simulink model "Ejercicio_2_DB"  (R2023a)
settings: Solver=VariableStepAuto  StartTime=0.0  StopTime=.5  RelTol=1e-6
values from neighbouring files (symbols this model uses):
  C3 = 10e-6    (= 1e-05)    [Ejercicio_2.m]
  C5 = C3    (= 1e-05)    [Ejercicio_2.m]
  G0 = 1/(C*inv(B*K-A)*B)    [Ejercicio_2.m]
  G1 = 1/R1    (= 0.001)    [Ejercicio_2.m]
  G2 = 1/R2    (= 0.001)    [Ejercicio_2.m]
  G4 = 1/R4    (= 0.0005)    [Ejercicio_2.m]
  G6a = 1/R6a    (= 0.001)    [Ejercicio_2.m]
  G6b = 1/R6b    (= 0.001)    [Ejercicio_2.m]
  K = acker(A,B,P_LC)    [Ejercicio_2.m]
settings Model: Creator=54115  LastModifiedBy=franc
settings SolverCC: AlgebraicLoopSolver=TrustRegion
settings DebuggingCC: UnconnectedInputMsg=warning  UnconnectedOutputMsg=warning  UnconnectedLineMsg=warning
settings ModelReferenceCC: EnableRefExpFcnMdlSchedulingChecks=on

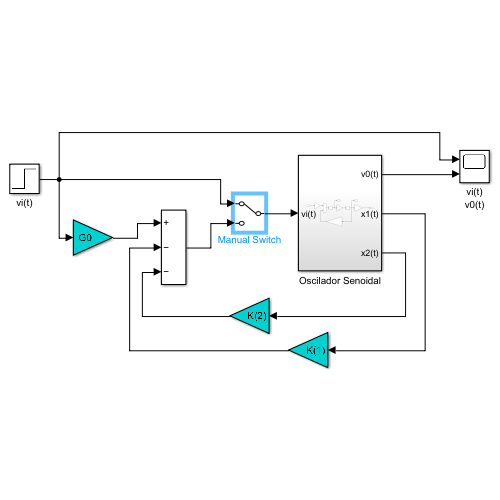
[thumbnail: Simulink's stored preview of the top-level diagram]
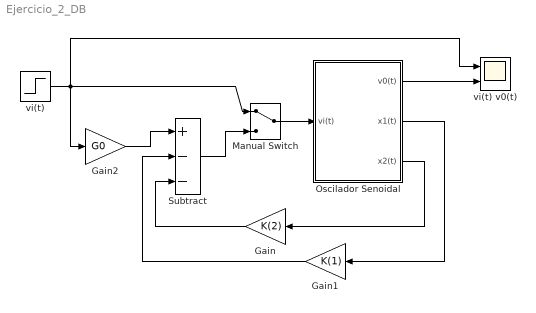
== system Ejercicio_2_DB ==
  Gain : Gain  Gain=K(2)
  Gain1 : Gain  Gain=K(1)
  Gain2 : Gain  Gain=G0
  Manual Switch : ManualSwitch
  Oscilador Senoidal : Subsystem
  Subtract : Sum  Inputs=+--
  vi(t) : Step  Time=0  SampleTime=0
  vi(t) v0(t) : Scope  NumInputPorts=2
  wires:
  Gain/1 -> Subtract/3
  Gain1/1 -> Subtract/2
  vi(t)/1 -> Gain2/1, Manual Switch/1, vi(t) v0(t)/1
  Gain2/1 -> Subtract/1
  Oscilador Senoidal/3(x2(t)) -> Gain/1
  Oscilador Senoidal/2(x1(t)) -> Gain1/1
  Oscilador Senoidal/1(v0(t)) -> vi(t) v0(t)/2
  Manual Switch/1 -> Oscilador Senoidal/1(vi(t))
  Subtract/1 -> Manual Switch/2

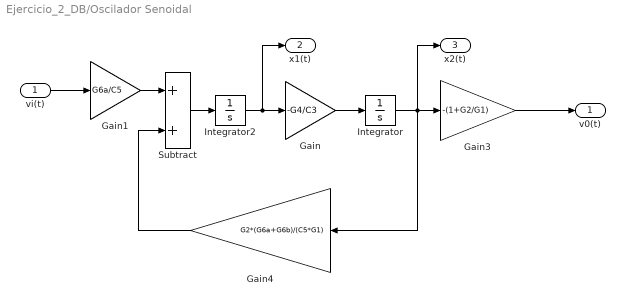
== system Ejercicio_2_DB/Oscilador Senoidal ==
  vi(t) : Inport
  Gain : Gain  Gain=-G4/C3
  Gain1 : Gain  Gain=G6a/C5
  Gain3 : Gain  Gain=-(1+G2/G1)
  Gain4 : Gain  Gain=G2*(G6a+G6b)/(C5*G1)
  Integrator : Integrator
  Integrator2 : Integrator
  Subtract : Sum
  v0(t) : Outport
  x1(t) : Outport  Port=2
  x2(t) : Outport  Port=3
  wires:
  vi(t)/1 -> Gain1/1
  Gain1/1 -> Subtract/1
  Integrator/1 -> x2(t)/1, Gain3/1, Gain4/1
  Gain4/1 -> Subtract/2
  Gain3/1 -> v0(t)/1
  Gain/1 -> Integrator/1
  Integrator2/1 -> x1(t)/1, Gain/1
  Subtract/1 -> Integrator2/1
